simulink library "EnergyConverters"  (R2023a)
settings: Solver=VariableStepAuto  StartTime=0.0  StopTime=10.0  RelTol=1e-3
undefined symbols (not defined in the file or in its folder): delta_h_C_air, eta_EG_map, eta_EM_mapG, eta_EM_mapM, h, H_o_m, H_u, i_FC_in, i_FC_max, k1, k2, k3, k4, M_air, P_CE_idle, T_CE_max, T_EG_max, T_EM_max, theta_CE, theta_EM, V_CE_map, V_FC_out, w_CE_idle, w_CE_max, w_CE_upper, w_EG_row, w_EG_upper, w_EM_row, w_EM_upper
settings Model: Creator=dadikozyanaa  LastModifiedBy=bestt
settings OptimizationCC: ReuseModelBlockBuffer=off
settings DebuggingCC: UnconnectedInputMsg=warning  UnconnectedOutputMsg=warning  UnconnectedLineMsg=warning
settings ModelReferenceCC: EnableRefExpFcnMdlSchedulingChecks=on
settings RTWCC: DLArmComputeVersion=19.05

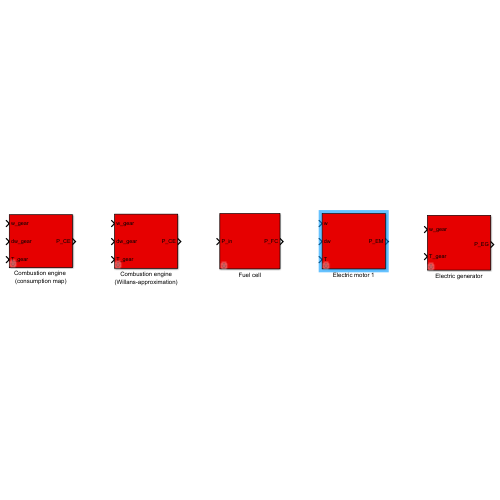
[thumbnail: Simulink's stored preview of the top-level diagram]
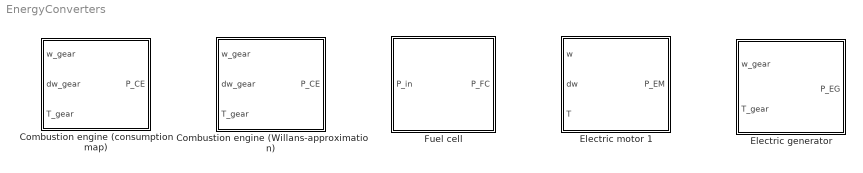
== system EnergyConverters ==
  Combustion engine (Willans-approximation) : Subsystem  Tag=combustion engine  mask(Combustion Engine (based on Willans approximation)){engine_type=Otto, V_d=0.708, theta_CE=0.05, S=50, B=45, w_CE_idle=105, P_CE_idle=2600, P_aux=300, e=0.46, PI=2, p_me0g=1, ENABLE_FUEL_CUTOFF=on, T_CE_cutoff=5, P_CE_cutoff=0}
      mask prompts: engine_type "Engine type"; V_d "Displacement [l]"; theta_CE "Engine inertia [kg*m^2]"; S "Stroke [mm]"; B "Bore diameter [mm]"; w_CE_idle "Engine speed at idle [rad/s]"; P_CE_idle "Engine power at idle [W]"; P_aux "Power required by auxiliaries  [W]"; e "1. Willans parameter: Engine internal thermodynamic efficiency [-]"; PI "2. Willans parameter: Maximum boost ratio [-]"; p_me0g "3. Willans parameter: Gas exchange losses [bar]"; ENABLE_FUEL_CUTOFF "Enable fuel cutoff"; T_CE_cutoff "Engine torque at fuel cutoff [Nm]"; P_CE_cutoff "Power at fuel cutoff [W]"
      mask help:
      | This block simulates the behaviour of a combustion engine. The block is based on the Willans approximation with friction part based on the ETH model.
      |
      | Input:
      | =====
      | 	w_gear	Speed of the fly wheel [rad/s]
      | 	dw_gear	Acceleration of the fly wheel [rad/s^2]
      | 	T_gear	Torque on the fly wheel [Nm]
      |
      | Output:
      | ======
      | 	P_CE	Power produced by the combustion engine [W]
      mask init:
      | init_CE_willans;
      mask TypeOptions engine_type: Otto | Diesel
  Combustion engine (consumption map) : Subsystem  Tag=combustion engine  mask(Combustion Engine (based on consumption map)){enginetype=Compression ignition, enginenumberCI=37kW, enginenumberSI=30kW, P_aux=0, ENABLE_FUEL_CUTOFF=on, T_CE_cutoff=5, P_CE_cutoff=0, scale_CE=1}
      mask prompts: enginetype "Select an engine type"; enginenumberCI "Select an engine model"; enginenumberSI "Select an engine model"; P_aux "Power required by auxiliaries [W]"; ENABLE_FUEL_CUTOFF "Enable fuel cutoff"; T_CE_cutoff "Engine torque at fuel cutoff [Nm]"; P_CE_cutoff "Power at fuel cutoff [W]"; scale_CE "Engine scaling factor [-]"
      mask help:
      | This block simulates the behaviour of a combustion engine. The block is based on a consumption map.
      |
      | Input:
      | =====
      | 	w_gear	Speed of the fly wheel [rad/s]
      | 	dw_gear	Acceleration of the fly wheel [rad/s^2]
      | 	T_gear	Torque on the fly wheel [Nm]
      |
      | Output:
      | ======
      | 	P_CE	Power produced by the combustion engine [W]
      mask init:
      | init_CE_map;
      mask Help: web(which('help_CombustionEngineMap.html'), '-helpbrowser')
      mask TypeOptions enginetype: Compression ignition | Spark ignition
      mask Callback enginetype:
      | maskStr = get_param(gcb,'enginetype');
      | 
      | switch maskStr
      |     case 'Compression ignition'
      |         set_param(gcb,'MaskVisibilities',{'on';'on';'off';'on';'on';'on';'on';'on'}),
      |     case 'Spark ignition'
      |         set_param(gcb,'MaskVisibilities',{'on';'off';'on';'on';'on';'on';'on';'on'}),
      | end
      mask TypeOptions enginenumberCI: 37kW | 54kW | 67kW | 88kW | 119kW | 171kW | 205kW | 246kW | 330kW
      mask TypeOptions enginenumberSI: 30kW | 41kW | 95kW | 102kW | 186kW | 224kW
      mask DialogControl ParameterGroupVar Prompt: Engine type and model
      mask DialogControl Container3 Prompt: Parameters
  Electric generator : Subsystem  mask(Electric Generator){gentype=Permanent magnet, gennumberPM=32 kW, genenumberCE=92 %, scale_EG=1}
      mask prompts: gentype "Select an electric generator type:"; gennumberPM "Select an electric generator model:"; genenumberCE "Select an electric generator model:"; scale_EG "Generator scaling factor [-]:"
      mask help:
      | This block simulates the behaviour of an electric generator. The block is based on an efficiency map.
      |
      | Input:
      | =====
      | 	w_gear	Speed of the fly wheel [rad/s]
      | 	T_gear	Torque on the fly wheel [Nm]
      |
      | Output:
      | ======
      | 	P_EG	Power of the electric generator [W]
      mask init:
      | init_EG;
      mask TypeOptions gentype: Permanent magnet | Constant efficiency
      mask Callback gentype:
      | maskStr = get_param(gcb,'gentype');
      | 
      | switch maskStr
      |     case 'Permanent magnet'
      |         set_param(gcb,'MaskVisibilities',{'on';'on';'off';'on'}),
      |     case 'Constant efficiency'
      |         set_param(gcb,'MaskVisibilities',{'on';'off';'on';'on'}),
      | end
      mask TypeOptions gennumberPM: 15 kW | 32 kW | 63 kW
      mask TypeOptions genenumberCE: 92 % | 95 %
      mask DialogControl ParameterGroupVar Prompt: EG model and type
      mask DialogControl Container3 Prompt: Parameters
  Electric motor 1 : Subsystem  mask(Electric Motor){motortype=Permanet magnet, motornumberPM=8 kW, motornumberAC=25 kW, scale_EM=1, P_aux=100, motornumberSim=1}
      mask prompts: motortype "Select electric machine type:"; motornumberPM "Select electric machine model:"; motornumberAC "Select electric machine model:"; scale_EM "Motor scaling factor [-]:"; P_aux "Auxiliary power [W]:"; motornumberSim "Select electric machine number:"
      mask help:
      | This block simulates the behaviour of an electric motor. The block is based on an efficiency map.
      |
      | Input:
      | =====
      | 	w_gear	Speed of the fly wheel [rad/s]
      | 	dw_gear	Acceleration of the fly wheel [rad/s^2]
      | 	T_gear	Torque on the fly wheel [Nm]
      |
      | Output:
      | ======
      | 	P_EM	Power produced by the EM [W]
      mask init:
      | init_EM;
      mask Help: web(which('help_ElectricMotor.html'), '-helpbrowser')
      mask TypeOptions motortype: Permanet magnet | Induction (AC)
      mask Callback motortype:
      | maskStr = get_param(gcb,'motortype');
      | 
      | switch maskStr
      |     case 'Permanet magnet'
      |         set_param(gcb,'MaskVisibilities',{'on';'on';'off';'on';'on';'on'}),
      |     case 'Induction (AC)'
      |         set_param(gcb,'MaskVisibilities',{'on';'off';'on';'on';'on';'on'}),
      | end
      mask TypeOptions motornumberPM: 8 kW | 15 kW LYNX | 16 kW | 16 kW EVS | 25 kW | 30 kW Prius | 32 kW | 32 kW EV | 32 kW EVS | 33 kW | 49 kW | 58 kW | 100 kW
      mask TypeOptions motornumberAC: 25 kW | 30 kW | 59 kW | 62 kW | 75 kW | 83 kW | 124 kW | 150 kW | 187 kW
      mask TypeOptions motornumberSim: 1 | 2 | 3 | 4 | 5 | 6 | 7 | 8
      mask DialogControl ParameterGroupVar Prompt: EM type and model
      mask DialogControl Container3 Prompt: Parameters
      mask DialogControl ParameterGroupVar_copy Prompt: EM number
      mask Display:
      | %disp(messageEM, 'texmode', 'on')
      | %plot(w_EM_max, T_EM_max);
  Fuel cell : Subsystem  Tag=fuelcell  mask(Fuel Cell){N_FC=880, A_FC=190 * 1e-4, V_th=1.2, P_FC_idle=2000, eta_EM_C=0.75, eta_C=0.7, pi_C=1.3, T_air=25, l_air=1.5}
      mask prompts: N_FC "Number of fuel cells per stack (series connection) [-]"; A_FC "Size of fuel cell [m^2]"; V_th "Theoretical fuel cell voltage [V]"; P_FC_idle "Idle power [W]"; eta_EM_C "E-motor for air compressor efficiency [-]"; eta_C "Air compressor efficiency [-]"; pi_C "Air compression ratio [-]"; T_air "Air temperature [°C]"; l_air "Air to fuel ratio [-]"
      mask help:
      | This block simulates a fuel cell and converts fuel into electric energy.
      |
      | Input:
      | =====
      | 	P_in		Power required by the fuel cell [W]
      |
      | Output:
      | ======
      | 	P_FC		Power produced by the fuel cell [W]
      mask init:
      | init_FC;

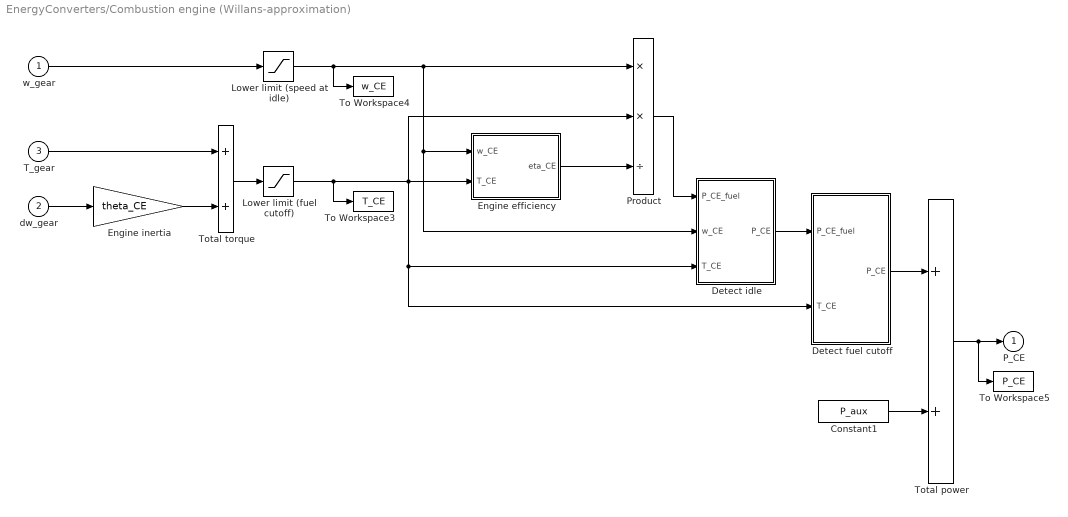
== system EnergyConverters/Combustion engine (Willans-approximation) ==
  w_gear : Inport
  dw_gear : Inport  Port=2
  T_gear : Inport  Port=3
  Constant1 : Constant  Value=P_aux
  Detect fuel cutoff : Subsystem  AncestorBlock=|
      | qss_tb_library/Energy Converter/Combustion Engine
      | (consumption map)/Detect fuel cutoff
      settings: LibrarySourceBlock=|
      | qss_tb_library/Energy Converter/Combustion Engine
      | (consumption map)/Detect fuel cutoff
  Detect idle : Subsystem
  Engine efficiency : Subsystem
  Engine inertia : Gain  Gain=theta_CE  SaturateOnIntegerOverflow=on  OutDataTypeStr=Inherit: Same as input  ParamDataTypeStr=Inherit: Same as input
  Lower limit (fuel cutoff) : Saturate  UpperLimit=inf  LowerLimit=T_CE_cutoff
  Lower limit (speed at idle) : Saturate  UpperLimit=inf  LowerLimit=w_CE_idle
  Product : Product  Inputs=**/  InputSameDT=on  RndMeth=Zero  SaturateOnIntegerOverflow=on  OutDataTypeStr=Inherit: Same as first input
  To Workspace3 : ToWorkspace  VariableName=T_CE  SampleTime=-1
  To Workspace4 : ToWorkspace  VariableName=w_CE  SampleTime=-1
  To Workspace5 : ToWorkspace  VariableName=P_CE  SampleTime=-1
  Total power : Sum  InputSameDT=on  SaturateOnIntegerOverflow=on  OutDataTypeStr=Inherit: Same as first input
  Total torque : Sum  InputSameDT=on  SaturateOnIntegerOverflow=on  OutDataTypeStr=Inherit: Same as first input
  P_CE : Outport  InitialOutput=0
  wires:
  Engine efficiency/1(eta_CE) -> Product/3
  T_gear/1 -> Total torque/1
  dw_gear/1 -> Engine inertia/1
  Total torque/1 -> Lower limit (fuel cutoff)/1
  Engine inertia/1 -> Total torque/2
  Lower limit (fuel cutoff)/1 -> Detect idle/3(T_CE), Detect fuel cutoff/2(T_CE), Engine efficiency/2(T_CE), Product/2, To Workspace3/1
  Lower limit (speed at idle)/1 -> To Workspace4/1, Engine efficiency/1(w_CE), Detect idle/2(w_CE), Product/1
  w_gear/1 -> Lower limit (speed at idle)/1
  Product/1 -> Detect idle/1(P_CE_fuel)
  Detect idle/1(P_CE) -> Detect fuel cutoff/1(P_CE_fuel)
  Detect fuel cutoff/1(P_CE) -> Total power/1
  Total power/1 -> P_CE/1, To Workspace5/1
  Constant1/1 -> Total power/2

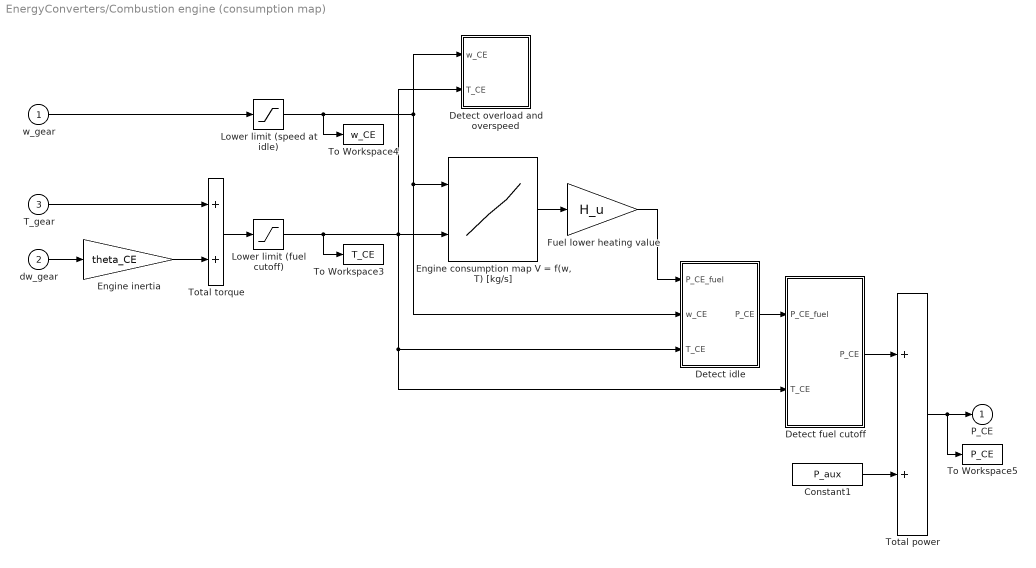
== system EnergyConverters/Combustion engine (consumption map) ==
  w_gear : Inport
  dw_gear : Inport  Port=2
  T_gear : Inport  Port=3
  Constant1 : Constant  Value=P_aux
  Detect fuel cutoff : Subsystem
  Detect idle : Subsystem
  Detect overload and overspeed : Subsystem
  "Engine consumption map V = f(w, T) [kg/s]" : Lookup2D  RowIndex=w_CE_row  ColumnIndex=T_CE_col  Table=V_CE_map  SaturateOnIntegerOverflow=off  InputSameDT=off
  Engine inertia : Gain  Gain=theta_CE  SaturateOnIntegerOverflow=on  OutDataTypeStr=Inherit: Same as input  ParamDataTypeStr=Inherit: Same as input
  Fuel lower heating value : Gain  Gain=H_u  SaturateOnIntegerOverflow=on  OutDataTypeStr=Inherit: Same as input  ParamDataTypeStr=Inherit: Same as input
  Lower limit (fuel cutoff) : Saturate  UpperLimit=inf  LowerLimit=T_CE_cutoff
  Lower limit (speed at idle) : Saturate  UpperLimit=inf  LowerLimit=w_CE_idle
  To Workspace3 : ToWorkspace  VariableName=T_CE  SampleTime=-1
  To Workspace4 : ToWorkspace  VariableName=w_CE  SampleTime=-1
  To Workspace5 : ToWorkspace  VariableName=P_CE  SampleTime=-1
  Total power : Sum  InputSameDT=on  SaturateOnIntegerOverflow=on  OutDataTypeStr=Inherit: Same as first input
  Total torque : Sum  InputSameDT=on  SaturateOnIntegerOverflow=on  OutDataTypeStr=Inherit: Same as first input
  P_CE : Outport  InitialOutput=0
  wires:
  Constant1/1 -> Total power/2
  Fuel lower heating value/1 -> Detect idle/1(P_CE_fuel)
  Total power/1 -> P_CE/1, To Workspace5/1
  Lower limit (fuel cutoff)/1 -> Detect overload and overspeed/2(T_CE), "Engine consumption map V = f(w, T) [kg/s]"/2, Detect idle/3(T_CE), Detect fuel cutoff/2(T_CE), To Workspace3/1
  Lower limit (speed at idle)/1 -> Detect overload and overspeed/1(w_CE), Detect idle/2(w_CE), "Engine consumption map V = f(w, T) [kg/s]"/1, To Workspace4/1
  "Engine consumption map V = f(w, T) [kg/s]"/1 -> Fuel lower heating value/1
  Detect fuel cutoff/1(P_CE) -> Total power/1
  T_gear/1 -> Total torque/1
  Total torque/1 -> Lower limit (fuel cutoff)/1
  Detect idle/1(P_CE) -> Detect fuel cutoff/1(P_CE_fuel)
  w_gear/1 -> Lower limit (speed at idle)/1
  Engine inertia/1 -> Total torque/2
  dw_gear/1 -> Engine inertia/1

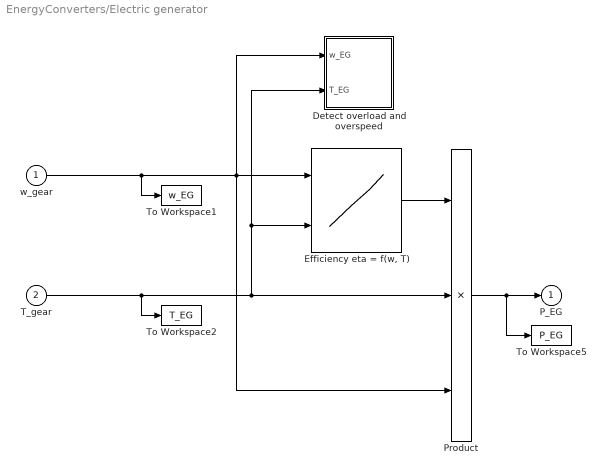
== system EnergyConverters/Electric generator ==
  w_gear : Inport
  T_gear : Inport  Port=2
  Detect overload and overspeed : Subsystem
  "Efficiency eta = f(w, T)" : Lookup2D  RowIndex=w_EG_row  ColumnIndex=T_EG_col  Table=eta_EG_map  SaturateOnIntegerOverflow=off  InputSameDT=off
  Product : Product  Inputs=3  InputSameDT=on  RndMeth=Zero  SaturateOnIntegerOverflow=on  OutDataTypeStr=Inherit: Same as first input
  To Workspace1 : ToWorkspace  VariableName=w_EG  SampleTime=-1
  To Workspace2 : ToWorkspace  VariableName=T_EG  SampleTime=-1
  To Workspace5 : ToWorkspace  VariableName=P_EG  SampleTime=-1
  P_EG : Outport  InitialOutput=0
  wires:
  T_gear/1 -> Product/2, "Efficiency eta = f(w, T)"/2, Detect overload and overspeed/2(T_EG), To Workspace2/1
  "Efficiency eta = f(w, T)"/1 -> Product/1
  Product/1 -> P_EG/1, To Workspace5/1
  w_gear/1 -> Product/3, "Efficiency eta = f(w, T)"/1, Detect overload and overspeed/1(w_EG), To Workspace1/1

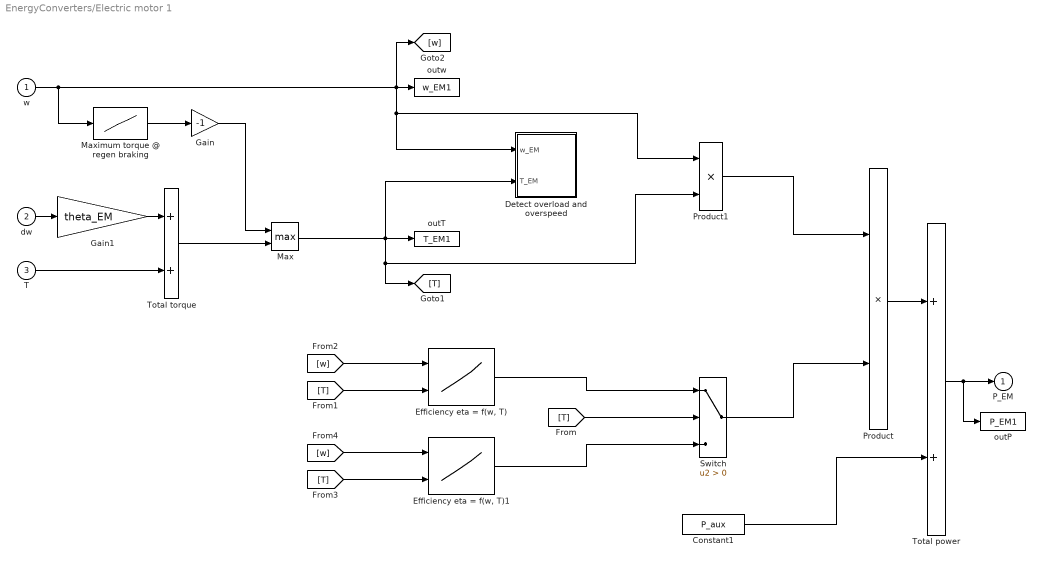
== system EnergyConverters/Electric motor 1 ==
  w : Inport
  dw : Inport  Port=2
  T : Inport  Port=3
  Constant1 : Constant  Value=P_aux
  Detect overload and overspeed : Subsystem
  "Efficiency eta = f(w, T)" : Lookup2D  RowIndex=w_EM_row  ColumnIndex=T_EM_col  Table=eta_EM_mapM  SaturateOnIntegerOverflow=off  InputSameDT=off
  "Efficiency eta = f(w, T)1" : Lookup2D  RowIndex=w_EM_row  ColumnIndex=T_EM_col  Table=eta_EM_mapG  SaturateOnIntegerOverflow=off  InputSameDT=off
  Gain : Gain  Gain=-1
  Gain1 : Gain  Gain=theta_EM  SaturateOnIntegerOverflow=on  OutDataTypeStr=Inherit: Same as input  ParamDataTypeStr=Inherit: Same as input
  Max : MinMax  Function=max  Inputs=2
  Maximum torque @ regen braking : Lookup  InputValues=w_EM_row  Table=T_EM_max
  Product : Product  InputSameDT=on  RndMeth=Zero  SaturateOnIntegerOverflow=on  OutDataTypeStr=Inherit: Same as first input
  Product1 : Product
  Switch : Switch  Criteria=u2 > Threshold  SaturateOnIntegerOverflow=off  InputSameDT=off
  Total power : Sum  InputSameDT=on  SaturateOnIntegerOverflow=on  OutDataTypeStr=Inherit: Same as first input
  Total torque : Sum  InputSameDT=on  SaturateOnIntegerOverflow=on  OutDataTypeStr=Inherit: Same as first input
  outP : ToWorkspace  VariableName=P_EM1  SampleTime=-1
  outT : ToWorkspace  VariableName=T_EM1  SampleTime=-1
  outw : ToWorkspace  VariableName=w_EM1  SampleTime=-1
  P_EM : Outport  InitialOutput=0
  wires:
  Total power/1 -> P_EM/1, outP/1
  Product/1 -> Total power/1
  Constant1/1 -> Total power/2
  Gain1/1 -> Total torque/1
  T/1 -> Total torque/2
  dw/1 -> Gain1/1
  w/1 -> Maximum torque @ regen braking/1, Product1/1, Detect overload and overspeed/1(w_EM), [w], outw/1
  [T] -> Switch/2
  "Efficiency eta = f(w, T)"/1 -> Switch/1
  "Efficiency eta = f(w, T)1"/1 -> Switch/3
  [w] -> "Efficiency eta = f(w, T)"/1
  [T] -> "Efficiency eta = f(w, T)"/2
  [w] -> "Efficiency eta = f(w, T)1"/1
  [T] -> "Efficiency eta = f(w, T)1"/2
  Product1/1 -> Product/1
  Switch/1 -> Product/2
  Maximum torque @ regen braking/1 -> Gain/1
  Total torque/1 -> Max/2
  Max/1 -> Detect overload and overspeed/2(T_EM), outT/1, Product1/2, [T]
  Gain/1 -> Max/1

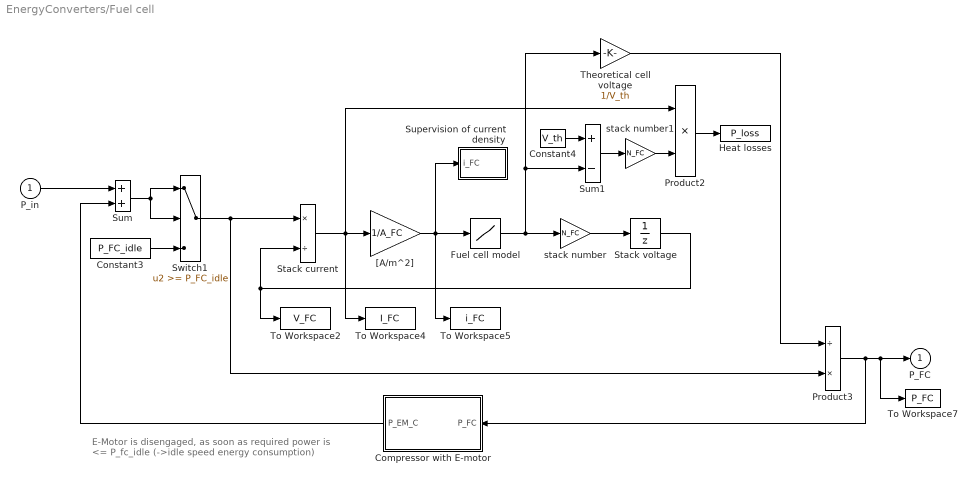
== system EnergyConverters/Fuel cell ==
  note: E-Motor is disengaged, as soon as required power
      |  is <= P_fc_idle (->idle speed energy consumption)
  P_in : Inport
  Compressor with E-motor : Subsystem
  Constant3 : Constant  Value=P_FC_idle
  Constant4 : Constant  Value=V_th
  Fuel cell model : Lookup  InputValues=i_FC_in  Table=V_FC_out
  Heat losses : ToWorkspace  VariableName=P_loss  SampleTime=1
  Product2 : Product  InputSameDT=on  RndMeth=Zero  SaturateOnIntegerOverflow=on  OutDataTypeStr=Inherit: Same as first input
  Product3 : Product  Inputs=/*  InputSameDT=on  RndMeth=Zero  SaturateOnIntegerOverflow=on  OutDataTypeStr=Inherit: Same as first input
  Stack current : Product  Inputs=*/  InputSameDT=on  RndMeth=Zero  SaturateOnIntegerOverflow=on  OutDataTypeStr=Inherit: Same as first input
  Stack voltage : UnitDelay  InitialCondition=10  SampleTime=h
  Sum : Sum  InputSameDT=on  SaturateOnIntegerOverflow=on  OutDataTypeStr=Inherit: Same as first input
  Sum1 : Sum  Inputs=+-  InputSameDT=on  SaturateOnIntegerOverflow=on  OutDataTypeStr=Inherit: Same as first input
  Supervision of current density : Subsystem
  Switch1 : Switch  Threshold=P_FC_idle
  Theoretical cell voltage : Gain  Gain=1/V_th  SaturateOnIntegerOverflow=on  OutDataTypeStr=Inherit: Same as input  ParamDataTypeStr=Inherit: Same as input
  To Workspace2 : ToWorkspace  VariableName=V_FC  SampleTime=1
  To Workspace4 : ToWorkspace  VariableName=I_FC  SampleTime=1
  To Workspace5 : ToWorkspace  VariableName=i_FC  SampleTime=1
  To Workspace7 : ToWorkspace  VariableName=P_FC  SampleTime=1
  "[A/m^2]" : Gain  Gain=1/A_FC  SaturateOnIntegerOverflow=on  OutDataTypeStr=Inherit: Same as input  ParamDataTypeStr=Inherit: Same as input
  stack number : Gain  Gain=N_FC  SaturateOnIntegerOverflow=on  OutDataTypeStr=Inherit: Same as input  ParamDataTypeStr=Inherit: Same as input
  stack number1 : Gain  Gain=N_FC  SaturateOnIntegerOverflow=on  OutDataTypeStr=Inherit: Same as input  ParamDataTypeStr=Inherit: Same as input
  P_FC : Outport  InitialOutput=0
  wires:
  Compressor with E-motor/1(P_EM_C) -> Sum/2
  Switch1/1 -> Stack current/1, Product3/2
  Constant3/1 -> Switch1/3
  Sum/1 -> Switch1/2, Switch1/1
  P_in/1 -> Sum/1
  Constant4/1 -> Sum1/1
  stack number/1 -> Stack voltage/1
  Sum1/1 -> stack number1/1
  stack number1/1 -> Product2/2
  "[A/m^2]"/1 -> Fuel cell model/1, To Workspace5/1, Supervision of current density/1("   i_FC")
  Theoretical cell voltage/1 -> Product3/1
  Fuel cell model/1 -> stack number/1, Sum1/2, Theoretical cell voltage/1
  Stack current/1 -> "[A/m^2]"/1, Product2/1, To Workspace4/1
  Stack voltage/1 -> Stack current/2, To Workspace2/1
  Product3/1 -> P_FC/1, To Workspace7/1, Compressor with E-motor/1(P_FC)
  Product2/1 -> Heat losses/1

== system EnergyConverters/Combustion engine (Willans-approximation)/Detect fuel cutoff ==
  P_CE_fuel : Inport
  T_CE : Inport  Port=2
  Constant1 : Constant  Value=ENABLE_FUEL_CUTOFF
  Constant3 : Constant  Value=P_CE_cutoff
  Decision : Switch  Threshold=0.5  SaturateOnIntegerOverflow=off  InputSameDT=off
  Detect fuel cutoff : Switch  Threshold=T_CE_cutoff + 0.01
  P_CE : Outport
  wires:
  Decision/1 -> P_CE/1
  Constant1/1 -> Decision/2
  Detect fuel cutoff/1 -> Decision/1
  P_CE_fuel/1 -> Decision/3, Detect fuel cutoff/1
  T_CE/1 -> Detect fuel cutoff/2
  Constant3/1 -> Detect fuel cutoff/3

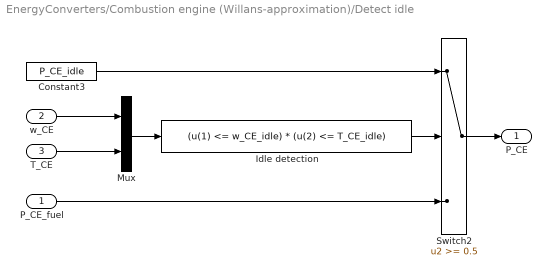
== system EnergyConverters/Combustion engine (Willans-approximation)/Detect idle ==
  P_CE_fuel : Inport
  w_CE : Inport  Port=2
  T_CE : Inport  Port=3
  Constant3 : Constant  Value=P_CE_idle
  Idle detection : Fcn  Expr=(u(1) <= w_CE_idle) * (u(2) <= T_CE_idle)
  Mux : Mux  Inputs=2
  Switch2 : Switch  Threshold=0.5
  P_CE : Outport  InitialOutput=0
  wires:
  Constant3/1 -> Switch2/1
  Switch2/1 -> P_CE/1
  P_CE_fuel/1 -> Switch2/3
  Idle detection/1 -> Switch2/2
  w_CE/1 -> Mux/1
  T_CE/1 -> Mux/2
  Mux/1 -> Idle detection/1

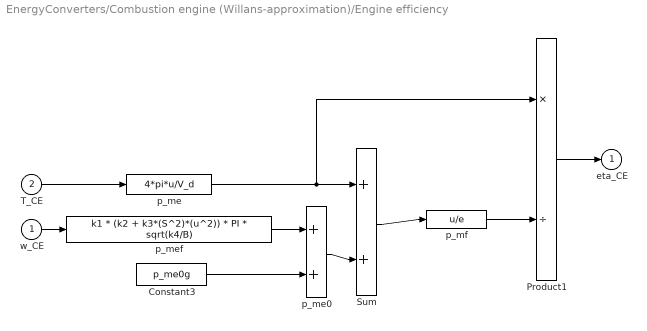
== system EnergyConverters/Combustion engine (Willans-approximation)/Engine efficiency ==
  w_CE : Inport
  T_CE : Inport  Port=2
  Constant3 : Constant  Value=p_me0g
  Product1 : Product  Inputs=*/  InputSameDT=on  RndMeth=Zero  SaturateOnIntegerOverflow=on  OutDataTypeStr=Inherit: Same as first input
  Sum : Sum  InputSameDT=on  SaturateOnIntegerOverflow=on  OutDataTypeStr=Inherit: Same as first input
  p_me : Fcn  Expr=4*pi*u/V_d
  p_me0 : Sum  InputSameDT=on  SaturateOnIntegerOverflow=on  OutDataTypeStr=Inherit: Same as first input
  p_mef : Fcn  Expr=k1 * (k2 + k3*(S^2)*(u^2)) * PI * sqrt(k4/B)
  p_mf : Fcn  Expr=u/e
  eta_CE : Outport  InitialOutput=0
  wires:
  Product1/1 -> eta_CE/1
  p_me/1 -> Sum/1, Product1/1
  Sum/1 -> p_mf/1
  p_mf/1 -> Product1/2
  p_me0/1 -> Sum/2
  T_CE/1 -> p_me/1
  w_CE/1 -> p_mef/1
  p_mef/1 -> p_me0/1
  Constant3/1 -> p_me0/2

== system EnergyConverters/Combustion engine (consumption map)/Detect fuel cutoff ==
  P_CE_fuel : Inport
  T_CE : Inport  Port=2
  Constant1 : Constant  Value=ENABLE_FUEL_CUTOFF
  Constant3 : Constant  Value=P_CE_cutoff
  Decision : Switch  Threshold=0.5  SaturateOnIntegerOverflow=off  InputSameDT=off
  Detect fuel cutoff : Switch  Threshold=T_CE_cutoff + 0.01
  P_CE : Outport
  wires:
  Constant3/1 -> Detect fuel cutoff/3
  T_CE/1 -> Detect fuel cutoff/2
  P_CE_fuel/1 -> Detect fuel cutoff/1, Decision/3
  Detect fuel cutoff/1 -> Decision/1
  Constant1/1 -> Decision/2
  Decision/1 -> P_CE/1

== system EnergyConverters/Combustion engine (consumption map)/Detect idle ==
  P_CE_fuel : Inport
  w_CE : Inport  Port=2
  T_CE : Inport  Port=3
  Constant3 : Constant  Value=P_CE_idle
  Idle detection : Fcn  Expr=(u(1) <= w_CE_idle) * (u(2) <= T_CE_idle)
  Mux : Mux  Inputs=2
  Switch2 : Switch  Threshold=0.5
  P_CE : Outport  InitialOutput=0
  wires:
  Mux/1 -> Idle detection/1
  T_CE/1 -> Mux/2
  w_CE/1 -> Mux/1
  Idle detection/1 -> Switch2/2
  P_CE_fuel/1 -> Switch2/3
  Switch2/1 -> P_CE/1
  Constant3/1 -> Switch2/1

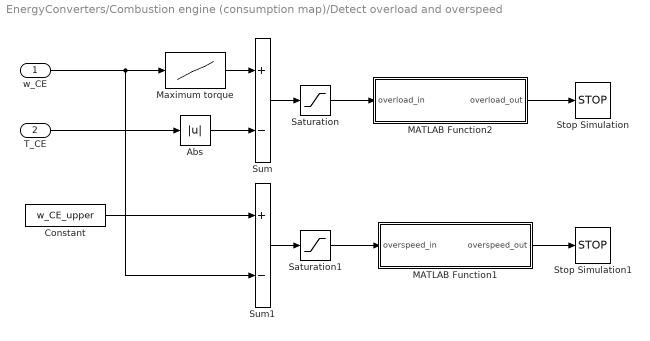
== system EnergyConverters/Combustion engine (consumption map)/Detect overload and overspeed ==
  w_CE : Inport
  T_CE : Inport  Port=2
  Abs : Abs
  Constant : Constant  Value=w_CE_upper
  MATLAB Function1 : MATLAB Function  TreatAsAtomicUnit=on
  MATLAB Function2 : MATLAB Function  TreatAsAtomicUnit=on
  Maximum torque : Lookup  InputValues=w_CE_max  Table=T_CE_max
  Saturation : Saturate  UpperLimit=0  LowerLimit=-inf
  Saturation1 : Saturate  UpperLimit=0  LowerLimit=-inf
  Stop Simulation : Stop
  Stop Simulation1 : Stop
  Sum : Sum  Inputs=+-  InputSameDT=on  SaturateOnIntegerOverflow=on  OutDataTypeStr=Inherit: Same as first input
  Sum1 : Sum  Inputs=+-  InputSameDT=on  SaturateOnIntegerOverflow=on  OutDataTypeStr=Inherit: Same as first input
  wires:
  Sum/1 -> Saturation/1
  w_CE/1 -> Maximum torque/1, Sum1/2
  T_CE/1 -> Abs/1
  Maximum torque/1 -> Sum/1
  Abs/1 -> Sum/2
  Constant/1 -> Sum1/1
  Sum1/1 -> Saturation1/1
  Saturation/1 -> MATLAB Function2/1(overload_in)
  MATLAB Function2/1(overload_out) -> Stop Simulation/1
  MATLAB Function1/1(overspeed_out) -> Stop Simulation1/1
  Saturation1/1 -> MATLAB Function1/1(overspeed_in)

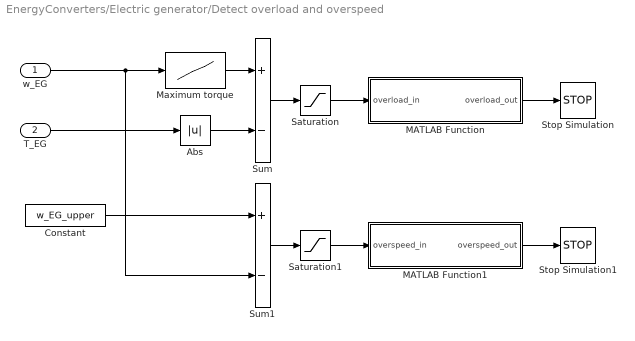
== system EnergyConverters/Electric generator/Detect overload and overspeed ==
  w_EG : Inport
  T_EG : Inport  Port=2
  Abs : Abs
  Constant : Constant  Value=w_EG_upper
  MATLAB Function : MATLAB Function  TreatAsAtomicUnit=on
  MATLAB Function1 : MATLAB Function  TreatAsAtomicUnit=on
  Maximum torque : Lookup  InputValues=w_EG_row  Table=T_EG_max
  Saturation : Saturate  UpperLimit=0  LowerLimit=-inf
  Saturation1 : Saturate  UpperLimit=0  LowerLimit=-inf
  Stop Simulation : Stop
  Stop Simulation1 : Stop
  Sum : Sum  Inputs=+-  InputSameDT=on  SaturateOnIntegerOverflow=on  OutDataTypeStr=Inherit: Same as first input
  Sum1 : Sum  Inputs=+-  InputSameDT=on  SaturateOnIntegerOverflow=on  OutDataTypeStr=Inherit: Same as first input
  wires:
  Sum/1 -> Saturation/1
  w_EG/1 -> Maximum torque/1, Sum1/2
  T_EG/1 -> Abs/1
  Maximum torque/1 -> Sum/1
  Abs/1 -> Sum/2
  Constant/1 -> Sum1/1
  Sum1/1 -> Saturation1/1
  Saturation/1 -> MATLAB Function/1(overload_in)
  MATLAB Function/1(overload_out) -> Stop Simulation/1
  Saturation1/1 -> MATLAB Function1/1(overspeed_in)
  MATLAB Function1/1(overspeed_out) -> Stop Simulation1/1

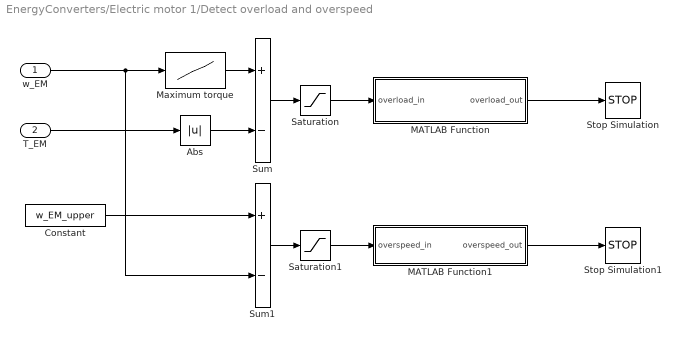
== system EnergyConverters/Electric motor 1/Detect overload and overspeed ==
  w_EM : Inport
  T_EM : Inport  Port=2
  Abs : Abs
  Constant : Constant  Value=w_EM_upper
  MATLAB Function : MATLAB Function  TreatAsAtomicUnit=on
  MATLAB Function1 : MATLAB Function  TreatAsAtomicUnit=on
  Maximum torque : Lookup  InputValues=w_EM_row  Table=T_EM_max
  Saturation : Saturate  UpperLimit=0  LowerLimit=-inf
  Saturation1 : Saturate  UpperLimit=0  LowerLimit=-inf
  Stop Simulation : Stop
  Stop Simulation1 : Stop
  Sum : Sum  Inputs=+-  InputSameDT=on  SaturateOnIntegerOverflow=on  OutDataTypeStr=Inherit: Same as first input
  Sum1 : Sum  Inputs=+-  InputSameDT=on  SaturateOnIntegerOverflow=on  OutDataTypeStr=Inherit: Same as first input
  wires:
  MATLAB Function1/1(overspeed_out) -> Stop Simulation1/1
  MATLAB Function/1(overload_out) -> Stop Simulation/1
  Sum/1 -> Saturation/1
  w_EM/1 -> Maximum torque/1, Sum1/2
  T_EM/1 -> Abs/1
  Maximum torque/1 -> Sum/1
  Abs/1 -> Sum/2
  Saturation/1 -> MATLAB Function/1(overload_in)
  Constant/1 -> Sum1/1
  Sum1/1 -> Saturation1/1
  Saturation1/1 -> MATLAB Function1/1(overspeed_in)

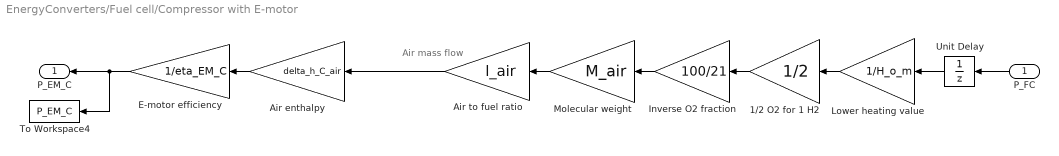
== system EnergyConverters/Fuel cell/Compressor with E-motor ==
  note: Air mass flow
  P_FC : Inport
  1/2 O2 for 1 H2 : Gain  Gain=1/2  SaturateOnIntegerOverflow=on  OutDataTypeStr=Inherit: Same as input  ParamDataTypeStr=Inherit: Same as input
  Air enthalpy : Gain  Gain=delta_h_C_air  SaturateOnIntegerOverflow=on  OutDataTypeStr=Inherit: Same as input  ParamDataTypeStr=Inherit: Same as input
  Air to fuel ratio : Gain  Gain=l_air  SaturateOnIntegerOverflow=on  OutDataTypeStr=Inherit: Same as input  ParamDataTypeStr=Inherit: Same as input
  E-motor efficiency : Gain  Gain=1/eta_EM_C  SaturateOnIntegerOverflow=on  OutDataTypeStr=Inherit: Same as input  ParamDataTypeStr=Inherit: Same as input
  Inverse O2 fraction : Gain  Gain=100/21  SaturateOnIntegerOverflow=on  OutDataTypeStr=Inherit: Same as input  ParamDataTypeStr=Inherit: Same as input
  Lower heating value : Gain  Gain=1/H_o_m  SaturateOnIntegerOverflow=on  OutDataTypeStr=Inherit: Same as input  ParamDataTypeStr=Inherit: Same as input
  Molecular weight : Gain  Gain=M_air  SaturateOnIntegerOverflow=on  OutDataTypeStr=Inherit: Same as input  ParamDataTypeStr=Inherit: Same as input
  To Workspace4 : ToWorkspace  VariableName=P_EM_C  SampleTime=1
  Unit Delay : UnitDelay  SampleTime=h
  P_EM_C : Outport  InitialOutput=0
  wires:
  Air enthalpy/1 -> E-motor efficiency/1
  Air to fuel ratio/1 -> Air enthalpy/1
  Unit Delay/1 -> Lower heating value/1
  Molecular weight/1 -> Air to fuel ratio/1
  Lower heating value/1 -> 1/2 O2 for 1 H2/1
  1/2 O2 for 1 H2/1 -> Inverse O2 fraction/1
  Inverse O2 fraction/1 -> Molecular weight/1
  E-motor efficiency/1 -> P_EM_C/1, To Workspace4/1
  P_FC/1 -> Unit Delay/1

== system EnergyConverters/Fuel cell/Supervision of current density ==
  "   i_FC" : Inport
  Constant6 : Constant  Value=i_FC_max
  MATLAB Function : MATLAB Function  TreatAsAtomicUnit=on
  Saturation1 : Saturate  UpperLimit=0  LowerLimit=-inf
  Stop Simulation : Stop
  Sum1 : Sum  Inputs=+-  InputSameDT=on  SaturateOnIntegerOverflow=on  OutDataTypeStr=Inherit: Same as first input
  wires:
  "   i_FC"/1 -> Sum1/2
  Constant6/1 -> Sum1/1
  Sum1/1 -> Saturation1/1
  MATLAB Function/1(overload_out) -> Stop Simulation/1
  Saturation1/1 -> MATLAB Function/1(overload_in)

== matlab function EnergyConverters/Electric motor 1/Detect overload and overspeed/MATLAB Function1 ==
  data: overspeed_in input; overspeed_out output
function overspeed_out = overspeed_fnc(overspeed_in)

if overspeed_in~=0
     disp('Simulation stopped due to Motor Overspeed.')
end

overspeed_out = overspeed_in;

== matlab function EnergyConverters/Electric generator/Detect overload and overspeed/MATLAB Function ==
  data: overload_in input; overload_out output
function overload_out = overload_fnc(overload_in)

if overload_in~=0
    disp('Simulation stopped due to Generator Overload.')
end

overload_out = overload_in;

== matlab function EnergyConverters/Electric generator/Detect overload and overspeed/MATLAB Function1 ==
  data: overspeed_in input; overspeed_out output
function overspeed_out = overspeed_fnc(overspeed_in)

if overspeed_in~=0
    disp('Simulation stopped due to Generator Overspeed.')
end

overspeed_out = overspeed_in;

== matlab function EnergyConverters/Fuel cell/Supervision of current density/MATLAB Function ==
  data: overload_in input; overload_out output
function overload_out = overload_fnc(overload_in)

if overload_in~=0
    disp('Simulation stopped due to Fuel Cell Current Overload.')
end

overload_out = overload_in;

== matlab function EnergyConverters/Combustion engine (consumption map)/Detect overload and overspeed/MATLAB Function1 ==
  data: overspeed_in input; overspeed_out output
function overspeed_out = overspeed_fnc(overspeed_in)

if overspeed_in~=0
    disp('Simulation stopped due to Engine Overspeed.')
end

overspeed_out = overspeed_in;

== matlab function EnergyConverters/Combustion engine (consumption map)/Detect overload and overspeed/MATLAB Function2 ==
  data: overload_in input; overload_out output
function overload_out = overload_fnc(overload_in)

if overload_in~=0
    disp('Simulation stopped due to Engine Overload.')
end

overload_out = overload_in;

== matlab function EnergyConverters/Electric motor 1/Detect overload and overspeed/MATLAB Function ==
  data: overload_in input; overload_out output
function overload_out = overload_fnc(overload_in)

if overload_in~=0
    disp('Simulation stopped due to Motor Overload.')
end

overload_out = overload_in;
